simulink model "controller_dev_sg_HIL_noTP"  (R2018b)
settings: configuration reference "Physics" (kept outside this file)
model workspace (MAT data in the model file):
  m = 1000
values from neighbouring files (symbols this model uses):
  bool_activate_Vehicles : value not decoded    [controller_dev_sg.sldd]
  ModObj_ObjList_SendPort = 11004.0    [UDPPortConfig.sldd]
  ModSens_GpsSenDat_SendPort = 3002.0    [UDPPortConfig.sldd]
  sensors_freq_camera = 37.0    [controller_dev_sg.sldd]
  sensors_freq_gps = 20.0    [controller_dev_sg.sldd]
  sensors_freq_imu = 100.0    [controller_dev_sg.sldd]
  sensors_freq_lidar = 12.0    [controller_dev_sg.sldd]
  sensors_freq_radar = 20.0    [controller_dev_sg.sldd]
undefined symbols (not defined in the file or in its folder): activate_VariableFriction, C, tpa_map_Reference, tSPhysics, x0_vehiclepos_start_veh1, x0_vehiclepos_start_veh10, x0_vehiclepos_start_veh2, x0_vehiclepos_start_veh3, x0_vehiclepos_start_veh4, x0_vehiclepos_start_veh5, x0_vehiclepos_start_veh6, x0_vehiclepos_start_veh7, x0_vehiclepos_start_veh8, x0_vehiclepos_start_veh9
libraries: xpcutilitieslib x273, xpcrtudplib x215, aerolibconvert2 x48, simulink x30, etargetslib x26, speedgoatlib_IO612 x7, canmsglib x6, slrtlib x4
(part 5 of 16)

== system controller_dev_sg_HIL_noTP/EnvironmentSim_Communication/prepare data for sending5 ==
  In1 : Inport
  Add : Sum
  Add1 : Sum
  Add2 : Sum
  Bus Selector1 : BusSelector  OutputSignals=x_m,y_m,z_m,phi_rad,theta_rad,psi_rad,nWheelFL_radps,DeltaWheel_rad,nWheelFR_radps,DeltaWheel_rad,nWheelRR_radps,nWheelRL_radps,ax_mps2,ay_mps2,az_mps2,dPhi_radps,dTheta_radps,dPsi_radps,x_m,y_m,psi_rad,vx_mps,vy_mps,nWheelFL_radps,nWheelFR_radps,nWheelRR_radps,nWheelRL_radps
  Clock : Clock
  Constant{,1..5} (6 alike) : Constant  Value=0
  Constant6 : Constant
  Constant7 : Constant  Value=pi
  Constant8 : Constant  Value=pi
  Gain : Gain  Gain=0.5
  Gain1 : Gain  Gain=0.5
  Integrator{,1..3} (4 alike) : Integrator
  Math Function : Math  Operator=square  SaturateOnIntegerOverflow=on
  Math Function1 : Math  Operator=square  SaturateOnIntegerOverflow=on
  Mux : Mux  Inputs=34
  Rate Transition{,1..26} (27 alike) : RateTransition
  Sqrt : Sqrt  SaturateOnIntegerOverflow=on
  normalieAngle1 : MATLAB Function  TreatAsAtomicUnit=on
  normalieAngle2 : MATLAB Function  TreatAsAtomicUnit=on
  Out1 : Outport
  wires:
  In1/1 -> Bus Selector1/1
  Bus Selector1/12 -> Integrator3/1  "<nWheelRL_radps>"
  Gain1/1 -> Add1/1
  Gain/1 -> Add2/2
  Bus Selector1/15 -> Rate Transition14/1  "<az_mps2>"
  Rate Transition22/1 -> Mux/31
  Constant7/1 -> Gain/1
  Bus Selector1/8 -> Rate Transition9/1  "<DeltaWheel_rad>"
  Bus Selector1/22 -> Math Function1/1  "<vx_mps>"
  Rate Transition12/1 -> Mux/20
  Rate Transition13/1 -> Mux/21
  Rate Transition17/1 -> Mux/25
  Sqrt/1 -> Rate Transition21/1
  Constant5/1 -> Mux/8
  Add1/1 -> normalieAngle2/1(u)
  Math Function1/1 -> Add/1
  Constant8/1 -> Gain1/1
  Rate Transition14/1 -> Mux/22
  Math Function/1 -> Add/2
  Bus Selector1/9 -> Integrator1/1  "<nWheelFR_radps>"
  Clock/1 -> Rate Transition26/1
  normalieAngle1/1(y) -> Rate Transition20/1
  Constant4/1 -> Mux/11
  Add2/1 -> normalieAngle1/1(u)
  Constant2/1 -> Mux/16
  Bus Selector1/6 -> Add1/2  "<psi_rad>"
  Constant6/1 -> Mux/29
  Rate Transition20/1 -> Mux/28
  Bus Selector1/24 -> Rate Transition22/1  "<nWheelFL_radps>"
  Integrator2/1 -> Rate Transition10/1
  Add/1 -> Sqrt/1
  Rate Transition23/1 -> Mux/32
  Rate Transition18/1 -> Mux/26
  Rate Transition26/1 -> Mux/1
  Rate Transition25/1 -> Mux/34
  Rate Transition8/1 -> Mux/13
  Bus Selector1/23 -> Math Function/1  "<vy_mps>"
  Bus Selector1/25 -> Rate Transition23/1  "<nWheelFR_radps>"
  Rate Transition10/1 -> Mux/15
  Constant/1 -> Mux/19
  Bus Selector1/20 -> Rate Transition19/1  "<y_m>"
  Rate Transition19/1 -> Mux/27
  Constant3/1 -> Mux/14
  Bus Selector1/21 -> Add2/1  "<psi_rad>"
  Integrator1/1 -> Rate Transition7/1
  Bus Selector1/26 -> Rate Transition24/1  "<nWheelRR_radps>"
  Rate Transition9/1 -> Mux/10
  Bus Selector1/18 -> Rate Transition17/1  "<dPsi_radps>"
  Bus Selector1/19 -> Rate Transition18/1  "<x_m>"
  Bus Selector1/13 -> Rate Transition12/1  "<ax_mps2>"
  Bus Selector1/17 -> Rate Transition16/1  "<dTheta_radps>"
  Integrator3/1 -> Rate Transition11/1
  Rate Transition15/1 -> Mux/23
  Rate Transition2/1 -> Mux/7
  Rate Transition16/1 -> Mux/24
  Bus Selector1/16 -> Rate Transition15/1  "<dPhi_radps>"
  Rate Transition6/1 -> Mux/9
  Rate Transition7/1 -> Mux/12
  Bus Selector1/11 -> Integrator2/1  "<nWheelRR_radps>"
  normalieAngle2/1(y) -> Rate Transition2/1
  Bus Selector1/27 -> Rate Transition25/1  "<nWheelRL_radps>"
  Rate Transition11/1 -> Mux/18
  Bus Selector1/14 -> Rate Transition13/1  "<ay_mps2>"
  Constant1/1 -> Mux/17
  Rate Transition5/1 -> Mux/4
  Rate Transition1/1 -> Mux/3
  Bus Selector1/3 -> Rate Transition5/1  "<z_m>"
  Bus Selector1/5 -> Rate Transition3/1  "<theta_rad>"
  Bus Selector1/2 -> Rate Transition1/1  "<y_m>"
  Bus Selector1/10 -> Rate Transition8/1  "<DeltaWheel_rad>"
  Bus Selector1/7 -> Integrator/1  "<nWheelFL_radps>"
  Bus Selector1/1 -> Rate Transition/1  "<x_m>"
  Integrator/1 -> Rate Transition6/1
  Rate Transition3/1 -> Mux/6
  Bus Selector1/4 -> Rate Transition4/1  "<phi_rad>"
  Rate Transition4/1 -> Mux/5
  Rate Transition21/1 -> Mux/30
  Rate Transition24/1 -> Mux/33
  Rate Transition/1 -> Mux/2
  Mux/1 -> Out1/1

== system controller_dev_sg_HIL_noTP/EnvironmentSim_Communication/prepare data for sending6 ==
  In1 : Inport
  Add : Sum
  Add1 : Sum
  Add2 : Sum
  Bus Selector1 : BusSelector  OutputSignals=x_m,y_m,z_m,phi_rad,theta_rad,psi_rad,nWheelFL_radps,DeltaWheel_rad,nWheelFR_radps,DeltaWheel_rad,nWheelRR_radps,nWheelRL_radps,ax_mps2,ay_mps2,az_mps2,dPhi_radps,dTheta_radps,dPsi_radps,x_m,y_m,psi_rad,vx_mps,vy_mps,nWheelFL_radps,nWheelFR_radps,nWheelRR_radps,nWheelRL_radps
  Clock : Clock
  Constant{,1..5} (6 alike) : Constant  Value=0
  Constant6 : Constant
  Constant7 : Constant  Value=pi
  Constant8 : Constant  Value=pi
  Gain : Gain  Gain=0.5
  Gain1 : Gain  Gain=0.5
  Integrator{,1..3} (4 alike) : Integrator
  Math Function : Math  Operator=square  SaturateOnIntegerOverflow=on
  Math Function1 : Math  Operator=square  SaturateOnIntegerOverflow=on
  Mux : Mux  Inputs=34
  Rate Transition{,1..26} (27 alike) : RateTransition
  Sqrt : Sqrt  SaturateOnIntegerOverflow=on
  normalieAngle1 : MATLAB Function  TreatAsAtomicUnit=on
  normalieAngle2 : MATLAB Function  TreatAsAtomicUnit=on
  Out1 : Outport
  wires:
  In1/1 -> Bus Selector1/1
  Bus Selector1/12 -> Integrator3/1  "<nWheelRL_radps>"
  Gain1/1 -> Add1/1
  Gain/1 -> Add2/2
  Bus Selector1/15 -> Rate Transition14/1  "<az_mps2>"
  Rate Transition22/1 -> Mux/31
  Constant7/1 -> Gain/1
  Bus Selector1/8 -> Rate Transition9/1  "<DeltaWheel_rad>"
  Bus Selector1/22 -> Math Function1/1  "<vx_mps>"
  Rate Transition12/1 -> Mux/20
  Rate Transition13/1 -> Mux/21
  Rate Transition17/1 -> Mux/25
  Sqrt/1 -> Rate Transition21/1
  Constant5/1 -> Mux/8
  Add1/1 -> normalieAngle2/1(u)
  Math Function1/1 -> Add/1
  Constant8/1 -> Gain1/1
  Rate Transition14/1 -> Mux/22
  Math Function/1 -> Add/2
  Bus Selector1/9 -> Integrator1/1  "<nWheelFR_radps>"
  Clock/1 -> Rate Transition26/1
  normalieAngle1/1(y) -> Rate Transition20/1
  Constant4/1 -> Mux/11
  Add2/1 -> normalieAngle1/1(u)
  Constant2/1 -> Mux/16
  Bus Selector1/6 -> Add1/2  "<psi_rad>"
  Constant6/1 -> Mux/29
  Rate Transition20/1 -> Mux/28
  Bus Selector1/24 -> Rate Transition22/1  "<nWheelFL_radps>"
  Integrator2/1 -> Rate Transition10/1
  Add/1 -> Sqrt/1
  Rate Transition23/1 -> Mux/32
  Rate Transition18/1 -> Mux/26
  Rate Transition26/1 -> Mux/1
  Rate Transition25/1 -> Mux/34
  Rate Transition8/1 -> Mux/13
  Bus Selector1/23 -> Math Function/1  "<vy_mps>"
  Bus Selector1/25 -> Rate Transition23/1  "<nWheelFR_radps>"
  Rate Transition10/1 -> Mux/15
  Constant/1 -> Mux/19
  Bus Selector1/20 -> Rate Transition19/1  "<y_m>"
  Rate Transition19/1 -> Mux/27
  Constant3/1 -> Mux/14
  Bus Selector1/21 -> Add2/1  "<psi_rad>"
  Integrator1/1 -> Rate Transition7/1
  Bus Selector1/26 -> Rate Transition24/1  "<nWheelRR_radps>"
  Rate Transition9/1 -> Mux/10
  Bus Selector1/18 -> Rate Transition17/1  "<dPsi_radps>"
  Bus Selector1/19 -> Rate Transition18/1  "<x_m>"
  Bus Selector1/13 -> Rate Transition12/1  "<ax_mps2>"
  Bus Selector1/17 -> Rate Transition16/1  "<dTheta_radps>"
  Integrator3/1 -> Rate Transition11/1
  Rate Transition15/1 -> Mux/23
  Rate Transition2/1 -> Mux/7
  Rate Transition16/1 -> Mux/24
  Bus Selector1/16 -> Rate Transition15/1  "<dPhi_radps>"
  Rate Transition6/1 -> Mux/9
  Rate Transition7/1 -> Mux/12
  Bus Selector1/11 -> Integrator2/1  "<nWheelRR_radps>"
  normalieAngle2/1(y) -> Rate Transition2/1
  Bus Selector1/27 -> Rate Transition25/1  "<nWheelRL_radps>"
  Rate Transition11/1 -> Mux/18
  Bus Selector1/14 -> Rate Transition13/1  "<ay_mps2>"
  Constant1/1 -> Mux/17
  Rate Transition5/1 -> Mux/4
  Rate Transition1/1 -> Mux/3
  Bus Selector1/3 -> Rate Transition5/1  "<z_m>"
  Bus Selector1/5 -> Rate Transition3/1  "<theta_rad>"
  Bus Selector1/2 -> Rate Transition1/1  "<y_m>"
  Bus Selector1/10 -> Rate Transition8/1  "<DeltaWheel_rad>"
  Bus Selector1/7 -> Integrator/1  "<nWheelFL_radps>"
  Bus Selector1/1 -> Rate Transition/1  "<x_m>"
  Integrator/1 -> Rate Transition6/1
  Rate Transition3/1 -> Mux/6
  Bus Selector1/4 -> Rate Transition4/1  "<phi_rad>"
  Rate Transition4/1 -> Mux/5
  Rate Transition21/1 -> Mux/30
  Rate Transition24/1 -> Mux/33
  Rate Transition/1 -> Mux/2
  Mux/1 -> Out1/1

== system controller_dev_sg_HIL_noTP/EnvironmentSim_Communication/prepare data for sending7 ==
  In1 : Inport
  Add : Sum
  Add1 : Sum
  Add2 : Sum
  Bus Selector1 : BusSelector  OutputSignals=x_m,y_m,z_m,phi_rad,theta_rad,psi_rad,nWheelFL_radps,DeltaWheel_rad,nWheelFR_radps,DeltaWheel_rad,nWheelRR_radps,nWheelRL_radps,ax_mps2,ay_mps2,az_mps2,dPhi_radps,dTheta_radps,dPsi_radps,x_m,y_m,psi_rad,vx_mps,vy_mps,nWheelFL_radps,nWheelFR_radps,nWheelRR_radps,nWheelRL_radps
  Clock : Clock
  Constant{,1..5} (6 alike) : Constant  Value=0
  Constant6 : Constant
  Constant7 : Constant  Value=pi
  Constant8 : Constant  Value=pi
  Gain : Gain  Gain=0.5
  Gain1 : Gain  Gain=0.5
  Integrator{,1..3} (4 alike) : Integrator
  Math Function : Math  Operator=square  SaturateOnIntegerOverflow=on
  Math Function1 : Math  Operator=square  SaturateOnIntegerOverflow=on
  Mux : Mux  Inputs=34
  Rate Transition{,1..26} (27 alike) : RateTransition
  Sqrt : Sqrt  SaturateOnIntegerOverflow=on
  normalieAngle1 : MATLAB Function  TreatAsAtomicUnit=on
  normalieAngle2 : MATLAB Function  TreatAsAtomicUnit=on
  Out1 : Outport
  wires:
  In1/1 -> Bus Selector1/1
  Bus Selector1/12 -> Integrator3/1  "<nWheelRL_radps>"
  Gain1/1 -> Add1/1
  Gain/1 -> Add2/2
  Bus Selector1/15 -> Rate Transition14/1  "<az_mps2>"
  Rate Transition22/1 -> Mux/31
  Constant7/1 -> Gain/1
  Bus Selector1/8 -> Rate Transition9/1  "<DeltaWheel_rad>"
  Bus Selector1/22 -> Math Function1/1  "<vx_mps>"
  Rate Transition12/1 -> Mux/20
  Rate Transition13/1 -> Mux/21
  Rate Transition17/1 -> Mux/25
  Sqrt/1 -> Rate Transition21/1
  Constant5/1 -> Mux/8
  Add1/1 -> normalieAngle2/1(u)
  Math Function1/1 -> Add/1
  Constant8/1 -> Gain1/1
  Rate Transition14/1 -> Mux/22
  Math Function/1 -> Add/2
  Bus Selector1/9 -> Integrator1/1  "<nWheelFR_radps>"
  Clock/1 -> Rate Transition26/1
  normalieAngle1/1(y) -> Rate Transition20/1
  Constant4/1 -> Mux/11
  Add2/1 -> normalieAngle1/1(u)
  Constant2/1 -> Mux/16
  Bus Selector1/6 -> Add1/2  "<psi_rad>"
  Constant6/1 -> Mux/29
  Rate Transition20/1 -> Mux/28
  Bus Selector1/24 -> Rate Transition22/1  "<nWheelFL_radps>"
  Integrator2/1 -> Rate Transition10/1
  Add/1 -> Sqrt/1
  Rate Transition23/1 -> Mux/32
  Rate Transition18/1 -> Mux/26
  Rate Transition26/1 -> Mux/1
  Rate Transition25/1 -> Mux/34
  Rate Transition8/1 -> Mux/13
  Bus Selector1/23 -> Math Function/1  "<vy_mps>"
  Bus Selector1/25 -> Rate Transition23/1  "<nWheelFR_radps>"
  Rate Transition10/1 -> Mux/15
  Constant/1 -> Mux/19
  Bus Selector1/20 -> Rate Transition19/1  "<y_m>"
  Rate Transition19/1 -> Mux/27
  Constant3/1 -> Mux/14
  Bus Selector1/21 -> Add2/1  "<psi_rad>"
  Integrator1/1 -> Rate Transition7/1
  Bus Selector1/26 -> Rate Transition24/1  "<nWheelRR_radps>"
  Rate Transition9/1 -> Mux/10
  Bus Selector1/18 -> Rate Transition17/1  "<dPsi_radps>"
  Bus Selector1/19 -> Rate Transition18/1  "<x_m>"
  Bus Selector1/13 -> Rate Transition12/1  "<ax_mps2>"
  Bus Selector1/17 -> Rate Transition16/1  "<dTheta_radps>"
  Integrator3/1 -> Rate Transition11/1
  Rate Transition15/1 -> Mux/23
  Rate Transition2/1 -> Mux/7
  Rate Transition16/1 -> Mux/24
  Bus Selector1/16 -> Rate Transition15/1  "<dPhi_radps>"
  Rate Transition6/1 -> Mux/9
  Rate Transition7/1 -> Mux/12
  Bus Selector1/11 -> Integrator2/1  "<nWheelRR_radps>"
  normalieAngle2/1(y) -> Rate Transition2/1
  Bus Selector1/27 -> Rate Transition25/1  "<nWheelRL_radps>"
  Rate Transition11/1 -> Mux/18
  Bus Selector1/14 -> Rate Transition13/1  "<ay_mps2>"
  Constant1/1 -> Mux/17
  Rate Transition5/1 -> Mux/4
  Rate Transition1/1 -> Mux/3
  Bus Selector1/3 -> Rate Transition5/1  "<z_m>"
  Bus Selector1/5 -> Rate Transition3/1  "<theta_rad>"
  Bus Selector1/2 -> Rate Transition1/1  "<y_m>"
  Bus Selector1/10 -> Rate Transition8/1  "<DeltaWheel_rad>"
  Bus Selector1/7 -> Integrator/1  "<nWheelFL_radps>"
  Bus Selector1/1 -> Rate Transition/1  "<x_m>"
  Integrator/1 -> Rate Transition6/1
  Rate Transition3/1 -> Mux/6
  Bus Selector1/4 -> Rate Transition4/1  "<phi_rad>"
  Rate Transition4/1 -> Mux/5
  Rate Transition21/1 -> Mux/30
  Rate Transition24/1 -> Mux/33
  Rate Transition/1 -> Mux/2
  Mux/1 -> Out1/1

== system controller_dev_sg_HIL_noTP/EnvironmentSim_Communication/prepare data for sending8 ==
  In1 : Inport
  Add : Sum
  Add1 : Sum
  Add2 : Sum
  Bus Selector1 : BusSelector  OutputSignals=x_m,y_m,z_m,phi_rad,theta_rad,psi_rad,nWheelFL_radps,DeltaWheel_rad,nWheelFR_radps,DeltaWheel_rad,nWheelRR_radps,nWheelRL_radps,ax_mps2,ay_mps2,az_mps2,dPhi_radps,dTheta_radps,dPsi_radps,x_m,y_m,psi_rad,vx_mps,vy_mps,nWheelFL_radps,nWheelFR_radps,nWheelRR_radps,nWheelRL_radps
  Clock : Clock
  Constant{,1..5} (6 alike) : Constant  Value=0
  Constant6 : Constant
  Constant7 : Constant  Value=pi
  Constant8 : Constant  Value=pi
  Gain : Gain  Gain=0.5
  Gain1 : Gain  Gain=0.5
  Integrator{,1..3} (4 alike) : Integrator
  Math Function : Math  Operator=square  SaturateOnIntegerOverflow=on
  Math Function1 : Math  Operator=square  SaturateOnIntegerOverflow=on
  Mux : Mux  Inputs=34
  Rate Transition{,1..26} (27 alike) : RateTransition
  Sqrt : Sqrt  SaturateOnIntegerOverflow=on
  normalieAngle1 : MATLAB Function  TreatAsAtomicUnit=on
  normalieAngle2 : MATLAB Function  TreatAsAtomicUnit=on
  Out1 : Outport
  wires:
  In1/1 -> Bus Selector1/1
  Bus Selector1/12 -> Integrator3/1  "<nWheelRL_radps>"
  Gain1/1 -> Add1/1
  Gain/1 -> Add2/2
  Bus Selector1/15 -> Rate Transition14/1  "<az_mps2>"
  Rate Transition22/1 -> Mux/31
  Constant7/1 -> Gain/1
  Bus Selector1/8 -> Rate Transition9/1  "<DeltaWheel_rad>"
  Bus Selector1/22 -> Math Function1/1  "<vx_mps>"
  Rate Transition12/1 -> Mux/20
  Rate Transition13/1 -> Mux/21
  Rate Transition17/1 -> Mux/25
  Sqrt/1 -> Rate Transition21/1
  Constant5/1 -> Mux/8
  Add1/1 -> normalieAngle2/1(u)
  Math Function1/1 -> Add/1
  Constant8/1 -> Gain1/1
  Rate Transition14/1 -> Mux/22
  Math Function/1 -> Add/2
  Bus Selector1/9 -> Integrator1/1  "<nWheelFR_radps>"
  Clock/1 -> Rate Transition26/1
  normalieAngle1/1(y) -> Rate Transition20/1
  Constant4/1 -> Mux/11
  Add2/1 -> normalieAngle1/1(u)
  Constant2/1 -> Mux/16
  Bus Selector1/6 -> Add1/2  "<psi_rad>"
  Constant6/1 -> Mux/29
  Rate Transition20/1 -> Mux/28
  Bus Selector1/24 -> Rate Transition22/1  "<nWheelFL_radps>"
  Integrator2/1 -> Rate Transition10/1
  Add/1 -> Sqrt/1
  Rate Transition23/1 -> Mux/32
  Rate Transition18/1 -> Mux/26
  Rate Transition26/1 -> Mux/1
  Rate Transition25/1 -> Mux/34
  Rate Transition8/1 -> Mux/13
  Bus Selector1/23 -> Math Function/1  "<vy_mps>"
  Bus Selector1/25 -> Rate Transition23/1  "<nWheelFR_radps>"
  Rate Transition10/1 -> Mux/15
  Constant/1 -> Mux/19
  Bus Selector1/20 -> Rate Transition19/1  "<y_m>"
  Rate Transition19/1 -> Mux/27
  Constant3/1 -> Mux/14
  Bus Selector1/21 -> Add2/1  "<psi_rad>"
  Integrator1/1 -> Rate Transition7/1
  Bus Selector1/26 -> Rate Transition24/1  "<nWheelRR_radps>"
  Rate Transition9/1 -> Mux/10
  Bus Selector1/18 -> Rate Transition17/1  "<dPsi_radps>"
  Bus Selector1/19 -> Rate Transition18/1  "<x_m>"
  Bus Selector1/13 -> Rate Transition12/1  "<ax_mps2>"
  Bus Selector1/17 -> Rate Transition16/1  "<dTheta_radps>"
  Integrator3/1 -> Rate Transition11/1
  Rate Transition15/1 -> Mux/23
  Rate Transition2/1 -> Mux/7
  Rate Transition16/1 -> Mux/24
  Bus Selector1/16 -> Rate Transition15/1  "<dPhi_radps>"
  Rate Transition6/1 -> Mux/9
  Rate Transition7/1 -> Mux/12
  Bus Selector1/11 -> Integrator2/1  "<nWheelRR_radps>"
  normalieAngle2/1(y) -> Rate Transition2/1
  Bus Selector1/27 -> Rate Transition25/1  "<nWheelRL_radps>"
  Rate Transition11/1 -> Mux/18
  Bus Selector1/14 -> Rate Transition13/1  "<ay_mps2>"
  Constant1/1 -> Mux/17
  Rate Transition5/1 -> Mux/4
  Rate Transition1/1 -> Mux/3
  Bus Selector1/3 -> Rate Transition5/1  "<z_m>"
  Bus Selector1/5 -> Rate Transition3/1  "<theta_rad>"
  Bus Selector1/2 -> Rate Transition1/1  "<y_m>"
  Bus Selector1/10 -> Rate Transition8/1  "<DeltaWheel_rad>"
  Bus Selector1/7 -> Integrator/1  "<nWheelFL_radps>"
  Bus Selector1/1 -> Rate Transition/1  "<x_m>"
  Integrator/1 -> Rate Transition6/1
  Rate Transition3/1 -> Mux/6
  Bus Selector1/4 -> Rate Transition4/1  "<phi_rad>"
  Rate Transition4/1 -> Mux/5
  Rate Transition21/1 -> Mux/30
  Rate Transition24/1 -> Mux/33
  Rate Transition/1 -> Mux/2
  Mux/1 -> Out1/1

== system controller_dev_sg_HIL_noTP/EnvironmentSim_Communication/prepare data for sending9 ==
  In1 : Inport
  Add : Sum
  Add1 : Sum
  Add2 : Sum
  Bus Selector1 : BusSelector  OutputSignals=x_m,y_m,z_m,phi_rad,theta_rad,psi_rad,nWheelFL_radps,DeltaWheel_rad,nWheelFR_radps,DeltaWheel_rad,nWheelRR_radps,nWheelRL_radps,ax_mps2,ay_mps2,az_mps2,dPhi_radps,dTheta_radps,dPsi_radps,x_m,y_m,psi_rad,vx_mps,vy_mps,nWheelFL_radps,nWheelFR_radps,nWheelRR_radps,nWheelRL_radps
  Clock : Clock
  Constant{,1..5} (6 alike) : Constant  Value=0
  Constant6 : Constant
  Constant7 : Constant  Value=pi
  Constant8 : Constant  Value=pi
  Gain : Gain  Gain=0.5
  Gain1 : Gain  Gain=0.5
  Integrator{,1..3} (4 alike) : Integrator
  Math Function : Math  Operator=square  SaturateOnIntegerOverflow=on
  Math Function1 : Math  Operator=square  SaturateOnIntegerOverflow=on
  Mux : Mux  Inputs=34
  Rate Transition{,1..26} (27 alike) : RateTransition
  Sqrt : Sqrt  SaturateOnIntegerOverflow=on
  normalieAngle1 : MATLAB Function  TreatAsAtomicUnit=on
  normalieAngle2 : MATLAB Function  TreatAsAtomicUnit=on
  Out1 : Outport
  wires:
  In1/1 -> Bus Selector1/1
  Bus Selector1/12 -> Integrator3/1  "<nWheelRL_radps>"
  Gain1/1 -> Add1/1
  Gain/1 -> Add2/2
  Bus Selector1/15 -> Rate Transition14/1  "<az_mps2>"
  Rate Transition22/1 -> Mux/31
  Constant7/1 -> Gain/1
  Bus Selector1/8 -> Rate Transition9/1  "<DeltaWheel_rad>"
  Bus Selector1/22 -> Math Function1/1  "<vx_mps>"
  Rate Transition12/1 -> Mux/20
  Rate Transition13/1 -> Mux/21
  Rate Transition17/1 -> Mux/25
  Sqrt/1 -> Rate Transition21/1
  Constant5/1 -> Mux/8
  Add1/1 -> normalieAngle2/1(u)
  Math Function1/1 -> Add/1
  Constant8/1 -> Gain1/1
  Rate Transition14/1 -> Mux/22
  Math Function/1 -> Add/2
  Bus Selector1/9 -> Integrator1/1  "<nWheelFR_radps>"
  Clock/1 -> Rate Transition26/1
  normalieAngle1/1(y) -> Rate Transition20/1
  Constant4/1 -> Mux/11
  Add2/1 -> normalieAngle1/1(u)
  Constant2/1 -> Mux/16
  Bus Selector1/6 -> Add1/2  "<psi_rad>"
  Constant6/1 -> Mux/29
  Rate Transition20/1 -> Mux/28
  Bus Selector1/24 -> Rate Transition22/1  "<nWheelFL_radps>"
  Integrator2/1 -> Rate Transition10/1
  Add/1 -> Sqrt/1
  Rate Transition23/1 -> Mux/32
  Rate Transition18/1 -> Mux/26
  Rate Transition26/1 -> Mux/1
  Rate Transition25/1 -> Mux/34
  Rate Transition8/1 -> Mux/13
  Bus Selector1/23 -> Math Function/1  "<vy_mps>"
  Bus Selector1/25 -> Rate Transition23/1  "<nWheelFR_radps>"
  Rate Transition10/1 -> Mux/15
  Constant/1 -> Mux/19
  Bus Selector1/20 -> Rate Transition19/1  "<y_m>"
  Rate Transition19/1 -> Mux/27
  Constant3/1 -> Mux/14
  Bus Selector1/21 -> Add2/1  "<psi_rad>"
  Integrator1/1 -> Rate Transition7/1
  Bus Selector1/26 -> Rate Transition24/1  "<nWheelRR_radps>"
  Rate Transition9/1 -> Mux/10
  Bus Selector1/18 -> Rate Transition17/1  "<dPsi_radps>"
  Bus Selector1/19 -> Rate Transition18/1  "<x_m>"
  Bus Selector1/13 -> Rate Transition12/1  "<ax_mps2>"
  Bus Selector1/17 -> Rate Transition16/1  "<dTheta_radps>"
  Integrator3/1 -> Rate Transition11/1
  Rate Transition15/1 -> Mux/23
  Rate Transition2/1 -> Mux/7
  Rate Transition16/1 -> Mux/24
  Bus Selector1/16 -> Rate Transition15/1  "<dPhi_radps>"
  Rate Transition6/1 -> Mux/9
  Rate Transition7/1 -> Mux/12
  Bus Selector1/11 -> Integrator2/1  "<nWheelRR_radps>"
  normalieAngle2/1(y) -> Rate Transition2/1
  Bus Selector1/27 -> Rate Transition25/1  "<nWheelRL_radps>"
  Rate Transition11/1 -> Mux/18
  Bus Selector1/14 -> Rate Transition13/1  "<ay_mps2>"
  Constant1/1 -> Mux/17
  Rate Transition5/1 -> Mux/4
  Rate Transition1/1 -> Mux/3
  Bus Selector1/3 -> Rate Transition5/1  "<z_m>"
  Bus Selector1/5 -> Rate Transition3/1  "<theta_rad>"
  Bus Selector1/2 -> Rate Transition1/1  "<y_m>"
  Bus Selector1/10 -> Rate Transition8/1  "<DeltaWheel_rad>"
  Bus Selector1/7 -> Integrator/1  "<nWheelFL_radps>"
  Bus Selector1/1 -> Rate Transition/1  "<x_m>"
  Integrator/1 -> Rate Transition6/1
  Rate Transition3/1 -> Mux/6
  Bus Selector1/4 -> Rate Transition4/1  "<phi_rad>"
  Rate Transition4/1 -> Mux/5
  Rate Transition21/1 -> Mux/30
  Rate Transition24/1 -> Mux/33
  Rate Transition/1 -> Mux/2
  Mux/1 -> Out1/1

== system controller_dev_sg_HIL_noTP/Subsystem4/ReadSteeringWheelInput ==
  Compare To Constant : simulink/Logic and Bit Operations/Compare To Constant  Priority=1  relop===  const=24  OutDataTypeStr=boolean
  Min. do-while count : Constant  OutDataTypeStr=int8  SampleTime=-1
  Subtrat : Sum  Inputs=+-
  UDP Receive : xpcrtudplib/UDP Receive  ipAddressVal=192.168.0.2  localPort=50004  rcvWidth=24  rcvFmAny=on  fmAddress=10.0.2.0  rcvMulticast=off  multicastAddress={}  maxUDPQueue=8  sampleTime=-1
      settings: SourceProductName=Simulink Real-Time
  While Iterator : WhileIterator  WhileBlockType=do-while  ShowIterationPort=on  OutputDataType=int16
  NumMsg : Outport
  Data : Outport  Port=2
  wires:
  Subtrat/1 -> NumMsg/1  "num msgs this timestep"
  UDP Receive/1 -> Data/1
  Min. do-while count/1 -> Subtrat/2
  While Iterator/1 -> Subtrat/1
  UDP Receive/2 -> Compare To Constant/1
  Compare To Constant/1 -> While Iterator/1

== system controller_dev_sg_HIL_noTP/Subsystem4/ReadSteeringWheelInputPackage ==
  Raw Data : Inport
  Enable : EnablePort
  Byte Unpack : etargetslib/Byte Unpack  dimensions={[1], [1], [1]}  datatypes={'double', 'double', 'double'}  byteAlign=1
  Terminator : Terminator
  Acceleration : Outport
  SteeringWheelAngle_rad : Outport  Port=2
  wires:
  Byte Unpack/1 -> Acceleration/1
  Byte Unpack/2 -> SteeringWheelAngle_rad/1
  Byte Unpack/3 -> Terminator/1
  Raw Data/1 -> Byte Unpack/1

== system controller_dev_sg_HIL_noTP/UDP from Control (Request for Steering Angle, Long. Force)/ReadControlCommands ==
  Compare To Constant : simulink/Logic and Bit Operations/Compare To Constant  relop===  const=40  OutDataTypeStr=boolean
  Min. do-while count : Constant  OutDataTypeStr=int8  SampleTime=-1
  Subtrat : Sum  Inputs=+-
  UDP Receive : xpcrtudplib/UDP Receive  ipAddressVal=10.0.0.20  localPort=ModCtrl_CtrlCommandVeh1_RcvPort  rcvWidth=40  rcvFmAny=on  fmAddress=10.0.0.1  rcvMulticast=off  multicastAddress={}  maxUDPQueue=8  sampleTime=-1
      settings: SourceProductName=Simulink Real-Time
  While Iterator : WhileIterator  WhileBlockType=do-while  ShowIterationPort=on  OutputDataType=int16
  Data : Outport
  NumMsg : Outport  Port=2
  wires:
  Compare To Constant/1 -> While Iterator/1
  UDP Receive/2 -> Compare To Constant/1
  While Iterator/1 -> Subtrat/1
  Min. do-while count/1 -> Subtrat/2
  Subtrat/1 -> NumMsg/1  "num msgs this timestep"
  UDP Receive/1 -> Data/1

== system controller_dev_sg_HIL_noTP/UDP from Control (Request for Steering Angle, Long. Force)/ReadControlCommandsPackage ==
  Raw Data : Inport
  Enable : EnablePort
  Byte Unpack : etargetslib/Byte Unpack  dimensions={[1], [1], [1], [1], [1]}  datatypes={'double', 'double', 'double', 'double', 'double'}  byteAlign=1
  Data Type Conversion{,1..4} (5 alike) : DataTypeConversion  OutDataTypeStr=double
  SteeringAngleRequest_rad : Outport
  LongForceRequest_N : Outport  Port=2
  ThrottleRequest_perc : Outport  Port=3
  GearRequest : Outport  Port=4
  BrakeRequest_bar : Outport  Port=5
  wires:
  Byte Unpack/1 -> Data Type Conversion/1
  Raw Data/1 -> Byte Unpack/1
  Byte Unpack/2 -> Data Type Conversion1/1
  Data Type Conversion/1 -> SteeringAngleRequest_rad/1
  Data Type Conversion1/1 -> LongForceRequest_N/1
  Byte Unpack/3 -> Data Type Conversion2/1
  Byte Unpack/4 -> Data Type Conversion3/1
  Byte Unpack/5 -> Data Type Conversion4/1
  Data Type Conversion2/1 -> ThrottleRequest_perc/1
  Data Type Conversion3/1 -> GearRequest/1
  Data Type Conversion4/1 -> BrakeRequest_bar/1

== system controller_dev_sg_HIL_noTP/UDP from Control (Request for Steering Angle, Long. Force)1/ReadControlCommands ==
  Compare To Constant : simulink/Logic and Bit Operations/Compare To Constant  relop===  const=40  OutDataTypeStr=boolean
  Min. do-while count : Constant  OutDataTypeStr=int8  SampleTime=-1
  Subtrat : Sum  Inputs=+-
  UDP Receive : xpcrtudplib/UDP Receive  ipAddressVal=10.0.0.20  localPort=ModCtrl_CtrlCommandVeh2_RcvPort  rcvWidth=40  rcvFmAny=on  fmAddress=10.0.0.1  rcvMulticast=off  multicastAddress={}  maxUDPQueue=8  sampleTime=-1
      settings: SourceProductName=Simulink Real-Time
  While Iterator : WhileIterator  WhileBlockType=do-while  ShowIterationPort=on  OutputDataType=int16
  Data : Outport
  NumMsg : Outport  Port=2
  wires:
  Compare To Constant/1 -> While Iterator/1
  UDP Receive/2 -> Compare To Constant/1
  While Iterator/1 -> Subtrat/1
  Min. do-while count/1 -> Subtrat/2
  Subtrat/1 -> NumMsg/1  "num msgs this timestep"
  UDP Receive/1 -> Data/1

== system controller_dev_sg_HIL_noTP/UDP from Control (Request for Steering Angle, Long. Force)1/ReadControlCommandsPackage ==
  Raw Data : Inport
  Enable : EnablePort
  Byte Unpack : etargetslib/Byte Unpack  dimensions={[1], [1], [1], [1], [1]}  datatypes={'double', 'double', 'double', 'double', 'double'}  byteAlign=1
  Data Type Conversion{,1..4} (5 alike) : DataTypeConversion  OutDataTypeStr=double
  SteeringAngleAtWheel_rad : Outport
  TractionForceSummedAtWheels_N : Outport  Port=2
  ThrottleRequest_perc : Outport  Port=3
  GearRequest : Outport  Port=4
  BrakeRequest_bar : Outport  Port=5
  wires:
  Byte Unpack/1 -> Data Type Conversion/1
  Raw Data/1 -> Byte Unpack/1
  Byte Unpack/2 -> Data Type Conversion1/1
  Data Type Conversion2/1 -> ThrottleRequest_perc/1
  Data Type Conversion4/1 -> BrakeRequest_bar/1
  Data Type Conversion/1 -> SteeringAngleAtWheel_rad/1
  Data Type Conversion1/1 -> TractionForceSummedAtWheels_N/1
  Data Type Conversion3/1 -> GearRequest/1
  Byte Unpack/3 -> Data Type Conversion2/1
  Byte Unpack/4 -> Data Type Conversion3/1
  Byte Unpack/5 -> Data Type Conversion4/1

== system controller_dev_sg_HIL_noTP/UDP from Control (Request for Steering Angle, Long. Force)2/ReadControlCommands ==
  Compare To Constant : simulink/Logic and Bit Operations/Compare To Constant  relop===  const=40  OutDataTypeStr=boolean
  Min. do-while count : Constant  OutDataTypeStr=int8  SampleTime=-1
  Subtrat : Sum  Inputs=+-
  UDP Receive : xpcrtudplib/UDP Receive  ipAddressVal=10.0.0.20  localPort=ModCtrl_CtrlCommandVeh3_RcvPort  rcvWidth=40  rcvFmAny=on  fmAddress=10.0.0.1  rcvMulticast=off  multicastAddress={}  maxUDPQueue=8  sampleTime=-1
      settings: SourceProductName=Simulink Real-Time
  While Iterator : WhileIterator  WhileBlockType=do-while  ShowIterationPort=on  OutputDataType=int16
  Data : Outport
  NumMsg : Outport  Port=2
  wires:
  Compare To Constant/1 -> While Iterator/1
  UDP Receive/2 -> Compare To Constant/1
  While Iterator/1 -> Subtrat/1
  Min. do-while count/1 -> Subtrat/2
  Subtrat/1 -> NumMsg/1  "num msgs this timestep"
  UDP Receive/1 -> Data/1

== system controller_dev_sg_HIL_noTP/UDP from Control (Request for Steering Angle, Long. Force)2/ReadControlCommandsPackage ==
  Raw Data : Inport
  Enable : EnablePort
  Byte Unpack : etargetslib/Byte Unpack  dimensions={[1], [1], [1], [1], [1]}  datatypes={'double', 'double', 'double', 'double', 'double'}  byteAlign=1
  Data Type Conversion{,1..2,4..5} (5 alike) : DataTypeConversion  OutDataTypeStr=double
  SteeringAngleAtWheel_rad : Outport
  TractionForceSummedAtWheels_N : Outport  Port=2
  ThrottleRequest_perc : Outport  Port=3
  GearRequest : Outport  Port=4
  BrakeRequest_bar : Outport  Port=5
  wires:
  Byte Unpack/1 -> Data Type Conversion/1
  Raw Data/1 -> Byte Unpack/1
  Byte Unpack/2 -> Data Type Conversion1/1
  Data Type Conversion2/1 -> ThrottleRequest_perc/1
  Data Type Conversion5/1 -> BrakeRequest_bar/1
  Data Type Conversion/1 -> SteeringAngleAtWheel_rad/1
  Data Type Conversion1/1 -> TractionForceSummedAtWheels_N/1
  Data Type Conversion4/1 -> GearRequest/1
  Byte Unpack/5 -> Data Type Conversion5/1
  Byte Unpack/4 -> Data Type Conversion4/1
  Byte Unpack/3 -> Data Type Conversion2/1

== system controller_dev_sg_HIL_noTP/UDP from Control (Request for Steering Angle, Long. Force)3/ReadControlCommands ==
  Compare To Constant : simulink/Logic and Bit Operations/Compare To Constant  relop===  const=40  OutDataTypeStr=boolean
  Min. do-while count : Constant  OutDataTypeStr=int8  SampleTime=-1
  Subtrat : Sum  Inputs=+-
  UDP Receive : xpcrtudplib/UDP Receive  ipAddressVal=10.0.0.20  localPort=ModCtrl_CtrlCommandVeh5_RcvPort  rcvWidth=40  rcvFmAny=on  fmAddress=10.0.0.1  rcvMulticast=off  multicastAddress={}  maxUDPQueue=8  sampleTime=-1
      settings: SourceProductName=Simulink Real-Time
  While Iterator : WhileIterator  WhileBlockType=do-while  ShowIterationPort=on  OutputDataType=int16
  Data : Outport
  NumMsg : Outport  Port=2
  wires:
  Compare To Constant/1 -> While Iterator/1
  UDP Receive/2 -> Compare To Constant/1
  While Iterator/1 -> Subtrat/1
  Min. do-while count/1 -> Subtrat/2
  Subtrat/1 -> NumMsg/1  "num msgs this timestep"
  UDP Receive/1 -> Data/1

== system controller_dev_sg_HIL_noTP/UDP from Control (Request for Steering Angle, Long. Force)3/ReadControlCommandsPackage ==
  Raw Data : Inport
  Enable : EnablePort
  Byte Unpack : etargetslib/Byte Unpack  dimensions={[1], [1], [1], [1], [1]}  datatypes={'double', 'double', 'double', 'double', 'double'}  byteAlign=1
  Data Type Conversion{,1..4} (5 alike) : DataTypeConversion  OutDataTypeStr=double
  SteeringAngleAtWheel_rad : Outport
  TractionForceSummedAtWheels_N : Outport  Port=2
  ThrottleRequest_perc : Outport  Port=3
  GearRequest : Outport  Port=4
  BrakeRequest_bar : Outport  Port=5
  wires:
  Byte Unpack/1 -> Data Type Conversion/1
  Raw Data/1 -> Byte Unpack/1
  Byte Unpack/2 -> Data Type Conversion1/1
  Byte Unpack/5 -> Data Type Conversion4/1
  Byte Unpack/4 -> Data Type Conversion3/1
  Byte Unpack/3 -> Data Type Conversion2/1
  Data Type Conversion2/1 -> ThrottleRequest_perc/1
  Data Type Conversion/1 -> SteeringAngleAtWheel_rad/1
  Data Type Conversion4/1 -> BrakeRequest_bar/1
  Data Type Conversion3/1 -> GearRequest/1
  Data Type Conversion1/1 -> TractionForceSummedAtWheels_N/1

== system controller_dev_sg_HIL_noTP/UDP from Control (Request for Steering Angle, Long. Force)4/ReadControlCommands ==
  Compare To Constant : simulink/Logic and Bit Operations/Compare To Constant  relop===  const=40  OutDataTypeStr=boolean
  Min. do-while count : Constant  OutDataTypeStr=int8  SampleTime=-1
  Subtrat : Sum  Inputs=+-
  UDP Receive : xpcrtudplib/UDP Receive  ipAddressVal=10.0.0.20  localPort=ModCtrl_CtrlCommandVeh4_RcvPort  rcvWidth=40  rcvFmAny=on  fmAddress=10.0.0.1  rcvMulticast=off  multicastAddress={}  maxUDPQueue=8  sampleTime=-1
      settings: SourceProductName=Simulink Real-Time
  While Iterator : WhileIterator  WhileBlockType=do-while  ShowIterationPort=on  OutputDataType=int16
  Data : Outport
  NumMsg : Outport  Port=2
  wires:
  Compare To Constant/1 -> While Iterator/1
  UDP Receive/2 -> Compare To Constant/1
  While Iterator/1 -> Subtrat/1
  Min. do-while count/1 -> Subtrat/2
  Subtrat/1 -> NumMsg/1  "num msgs this timestep"
  UDP Receive/1 -> Data/1

== system controller_dev_sg_HIL_noTP/UDP from Control (Request for Steering Angle, Long. Force)4/ReadControlCommandsPackage ==
  Raw Data : Inport
  Enable : EnablePort
  Byte Unpack : etargetslib/Byte Unpack  dimensions={[1], [1], [1], [1], [1]}  datatypes={'double', 'double', 'double', 'double', 'double'}  byteAlign=1
  Data Type Conversion{,1..4} (5 alike) : DataTypeConversion  OutDataTypeStr=double
  SteeringAngleAtWheel_rad : Outport
  TractionForceSummedAtWheels_N : Outport  Port=2
  ThrottleRequest_perc : Outport  Port=3
  GearRequest : Outport  Port=4
  BrakeRequest_bar : Outport  Port=5
  wires:
  Byte Unpack/1 -> Data Type Conversion/1
  Raw Data/1 -> Byte Unpack/1
  Byte Unpack/2 -> Data Type Conversion1/1
  Byte Unpack/5 -> Data Type Conversion4/1
  Byte Unpack/4 -> Data Type Conversion3/1
  Byte Unpack/3 -> Data Type Conversion2/1
  Data Type Conversion2/1 -> ThrottleRequest_perc/1
  Data Type Conversion/1 -> SteeringAngleAtWheel_rad/1
  Data Type Conversion4/1 -> BrakeRequest_bar/1
  Data Type Conversion3/1 -> GearRequest/1
  Data Type Conversion1/1 -> TractionForceSummedAtWheels_N/1

== system controller_dev_sg_HIL_noTP/UDP from Control (Request for Steering Angle, Long. Force)5/ReadControlCommands ==
  Compare To Constant : simulink/Logic and Bit Operations/Compare To Constant  relop===  const=40  OutDataTypeStr=boolean
  Min. do-while count : Constant  OutDataTypeStr=int8  SampleTime=-1
  Subtrat : Sum  Inputs=+-
  UDP Receive : xpcrtudplib/UDP Receive  ipAddressVal=10.0.0.20  localPort=ModCtrl_CtrlCommandVeh6_RcvPort  rcvWidth=40  rcvFmAny=on  fmAddress=10.0.0.1  rcvMulticast=off  multicastAddress={}  maxUDPQueue=8  sampleTime=-1
      settings: SourceProductName=Simulink Real-Time
  While Iterator : WhileIterator  WhileBlockType=do-while  ShowIterationPort=on  OutputDataType=int16
  Data : Outport
  NumMsg : Outport  Port=2
  wires:
  Compare To Constant/1 -> While Iterator/1
  UDP Receive/2 -> Compare To Constant/1
  While Iterator/1 -> Subtrat/1
  Min. do-while count/1 -> Subtrat/2
  Subtrat/1 -> NumMsg/1  "num msgs this timestep"
  UDP Receive/1 -> Data/1

== system controller_dev_sg_HIL_noTP/UDP from Control (Request for Steering Angle, Long. Force)5/ReadControlCommandsPackage ==
  Raw Data : Inport
  Enable : EnablePort
  Byte Unpack : etargetslib/Byte Unpack  dimensions={[1], [1], [1], [1], [1]}  datatypes={'double', 'double', 'double', 'double', 'double'}  byteAlign=1
  Data Type Conversion{,1..4} (5 alike) : DataTypeConversion  OutDataTypeStr=double
  SteeringAngleAtWheel_rad : Outport
  TractionForceSummedAtWheels_N : Outport  Port=2
  ThrottleRequest_perc : Outport  Port=3
  GearRequest : Outport  Port=4
  BrakeRequest_bar : Outport  Port=5
  wires:
  Byte Unpack/1 -> Data Type Conversion/1
  Raw Data/1 -> Byte Unpack/1
  Byte Unpack/2 -> Data Type Conversion1/1
  Byte Unpack/5 -> Data Type Conversion4/1
  Byte Unpack/4 -> Data Type Conversion3/1
  Byte Unpack/3 -> Data Type Conversion2/1
  Data Type Conversion2/1 -> ThrottleRequest_perc/1
  Data Type Conversion/1 -> SteeringAngleAtWheel_rad/1
  Data Type Conversion4/1 -> BrakeRequest_bar/1
  Data Type Conversion3/1 -> GearRequest/1
  Data Type Conversion1/1 -> TractionForceSummedAtWheels_N/1

== system controller_dev_sg_HIL_noTP/UDP from Control (Request for Steering Angle, Long. Force)6/ReadControlCommands ==
  Compare To Constant : simulink/Logic and Bit Operations/Compare To Constant  relop===  const=40  OutDataTypeStr=boolean
  Min. do-while count : Constant  OutDataTypeStr=int8  SampleTime=-1
  Subtrat : Sum  Inputs=+-
  UDP Receive : xpcrtudplib/UDP Receive  ipAddressVal=10.0.0.20  localPort=ModCtrl_CtrlCommandVeh7_RcvPort  rcvWidth=40  rcvFmAny=on  fmAddress=10.0.0.1  rcvMulticast=off  multicastAddress={}  maxUDPQueue=8  sampleTime=-1
      settings: SourceProductName=Simulink Real-Time
  While Iterator : WhileIterator  WhileBlockType=do-while  ShowIterationPort=on  OutputDataType=int16
  Data : Outport
  NumMsg : Outport  Port=2
  wires:
  Compare To Constant/1 -> While Iterator/1
  UDP Receive/2 -> Compare To Constant/1
  While Iterator/1 -> Subtrat/1
  Min. do-while count/1 -> Subtrat/2
  Subtrat/1 -> NumMsg/1  "num msgs this timestep"
  UDP Receive/1 -> Data/1

== system controller_dev_sg_HIL_noTP/UDP from Control (Request for Steering Angle, Long. Force)6/ReadControlCommandsPackage ==
  Raw Data : Inport
  Enable : EnablePort
  Byte Unpack : etargetslib/Byte Unpack  dimensions={[1], [1], [1], [1], [1]}  datatypes={'double', 'double', 'double', 'double', 'double'}  byteAlign=1
  Data Type Conversion{,1..4} (5 alike) : DataTypeConversion  OutDataTypeStr=double
  SteeringAngleAtWheel_rad : Outport
  TractionForceSummedAtWheels_N : Outport  Port=2
  ThrottleRequest_perc : Outport  Port=3
  GearRequest : Outport  Port=4
  BrakeRequest_bar : Outport  Port=5
  wires:
  Byte Unpack/1 -> Data Type Conversion/1
  Raw Data/1 -> Byte Unpack/1
  Byte Unpack/2 -> Data Type Conversion1/1
  Byte Unpack/5 -> Data Type Conversion4/1
  Byte Unpack/4 -> Data Type Conversion3/1
  Byte Unpack/3 -> Data Type Conversion2/1
  Data Type Conversion2/1 -> ThrottleRequest_perc/1
  Data Type Conversion/1 -> SteeringAngleAtWheel_rad/1
  Data Type Conversion4/1 -> BrakeRequest_bar/1
  Data Type Conversion3/1 -> GearRequest/1
  Data Type Conversion1/1 -> TractionForceSummedAtWheels_N/1

== system controller_dev_sg_HIL_noTP/UDP from Control (Request for Steering Angle, Long. Force)7/ReadControlCommands ==
  Compare To Constant : simulink/Logic and Bit Operations/Compare To Constant  relop===  const=40  OutDataTypeStr=boolean
  Min. do-while count : Constant  OutDataTypeStr=int8  SampleTime=-1
  Subtrat : Sum  Inputs=+-
  UDP Receive : xpcrtudplib/UDP Receive  ipAddressVal=10.0.0.20  localPort=ModCtrl_CtrlCommandVeh8_RcvPort  rcvWidth=40  rcvFmAny=on  fmAddress=10.0.0.1  rcvMulticast=off  multicastAddress={}  maxUDPQueue=8  sampleTime=-1
      settings: SourceProductName=Simulink Real-Time
  While Iterator : WhileIterator  WhileBlockType=do-while  ShowIterationPort=on  OutputDataType=int16
  Data : Outport
  NumMsg : Outport  Port=2
  wires:
  Compare To Constant/1 -> While Iterator/1
  UDP Receive/2 -> Compare To Constant/1
  While Iterator/1 -> Subtrat/1
  Min. do-while count/1 -> Subtrat/2
  Subtrat/1 -> NumMsg/1  "num msgs this timestep"
  UDP Receive/1 -> Data/1

== system controller_dev_sg_HIL_noTP/UDP from Control (Request for Steering Angle, Long. Force)7/ReadControlCommandsPackage ==
  Raw Data : Inport
  Enable : EnablePort
  Byte Unpack : etargetslib/Byte Unpack  dimensions={[1], [1], [1], [1], [1]}  datatypes={'double', 'double', 'double', 'double', 'double'}  byteAlign=1
  Data Type Conversion{,1..4} (5 alike) : DataTypeConversion  OutDataTypeStr=double
  SteeringAngleAtWheel_rad : Outport
  TractionForceSummedAtWheels_N : Outport  Port=2
  ThrottleRequest_perc : Outport  Port=3
  GearRequest : Outport  Port=4
  BrakeRequest_bar : Outport  Port=5
  wires:
  Byte Unpack/1 -> Data Type Conversion/1
  Raw Data/1 -> Byte Unpack/1
  Byte Unpack/2 -> Data Type Conversion1/1
  Byte Unpack/5 -> Data Type Conversion4/1
  Byte Unpack/4 -> Data Type Conversion3/1
  Byte Unpack/3 -> Data Type Conversion2/1
  Data Type Conversion2/1 -> ThrottleRequest_perc/1
  Data Type Conversion/1 -> SteeringAngleAtWheel_rad/1
  Data Type Conversion4/1 -> BrakeRequest_bar/1
  Data Type Conversion3/1 -> GearRequest/1
  Data Type Conversion1/1 -> TractionForceSummedAtWheels_N/1

== system controller_dev_sg_HIL_noTP/UDP to Object Detection/Prepare Object List1 ==
  Objects : Inport
  Bus Selector1 : BusSelector  OutputSignals=Object_1,Object_2,Object_3,Object_4,Object_5,Object_6,Object_7,Object_8,Object_9,Object_10
  Byte Pack : etargetslib/Byte Pack  datatypes={['double']}  byteAlign=1
  Data Type Conversion4 : DataTypeConversion
  Matrix Concatenate : Concatenate  NumInputs=10  Mode=Multidimensional array
  ObjList_Package : Outport
  wires:
  Byte Pack/1 -> ObjList_Package/1
  Data Type Conversion4/1 -> Byte Pack/1
  Objects/1 -> Bus Selector1/1
  Matrix Concatenate/1 -> Data Type Conversion4/1
  Bus Selector1/1 -> Matrix Concatenate/1  "<Object_1>"
  Bus Selector1/2 -> Matrix Concatenate/2  "<Object_2>"
  Bus Selector1/3 -> Matrix Concatenate/3  "<Object_3>"
  Bus Selector1/4 -> Matrix Concatenate/4  "<Object_4>"
  Bus Selector1/5 -> Matrix Concatenate/5  "<Object_5>"
  Bus Selector1/6 -> Matrix Concatenate/6  "<Object_6>"
  Bus Selector1/7 -> Matrix Concatenate/7  "<Object_7>"
  Bus Selector1/8 -> Matrix Concatenate/8  "<Object_8>"
  Bus Selector1/9 -> Matrix Concatenate/9  "<Object_9>"
  Bus Selector1/10 -> Matrix Concatenate/10  "<Object_10>"

== system controller_dev_sg_HIL_noTP/UDP to Object Detection/Prepare Object List10 ==
  Objects : Inport
  Bus Selector1 : BusSelector  OutputSignals=Object_1,Object_2,Object_3,Object_4,Object_5,Object_6,Object_7,Object_8,Object_9,Object_10
  Byte Pack : etargetslib/Byte Pack  datatypes={['double']}  byteAlign=1
  Data Type Conversion4 : DataTypeConversion
  Matrix Concatenate : Concatenate  NumInputs=10  Mode=Multidimensional array
  ObjList_Package : Outport
  wires:
  Byte Pack/1 -> ObjList_Package/1
  Data Type Conversion4/1 -> Byte Pack/1
  Objects/1 -> Bus Selector1/1
  Matrix Concatenate/1 -> Data Type Conversion4/1
  Bus Selector1/1 -> Matrix Concatenate/1  "<Object_1>"
  Bus Selector1/2 -> Matrix Concatenate/2  "<Object_2>"
  Bus Selector1/3 -> Matrix Concatenate/3  "<Object_3>"
  Bus Selector1/4 -> Matrix Concatenate/4  "<Object_4>"
  Bus Selector1/5 -> Matrix Concatenate/5  "<Object_5>"
  Bus Selector1/6 -> Matrix Concatenate/6  "<Object_6>"
  Bus Selector1/7 -> Matrix Concatenate/7  "<Object_7>"
  Bus Selector1/8 -> Matrix Concatenate/8  "<Object_8>"
  Bus Selector1/9 -> Matrix Concatenate/9  "<Object_9>"
  Bus Selector1/10 -> Matrix Concatenate/10  "<Object_10>"

== system controller_dev_sg_HIL_noTP/UDP to Object Detection/Prepare Object List2 ==
  Objects : Inport
  Bus Selector1 : BusSelector  OutputSignals=Object_1,Object_2,Object_3,Object_4,Object_5,Object_6,Object_7,Object_8,Object_9,Object_10
  Byte Pack : etargetslib/Byte Pack  datatypes={['double']}  byteAlign=1
  Data Type Conversion4 : DataTypeConversion
  Matrix Concatenate : Concatenate  NumInputs=10  Mode=Multidimensional array
  ObjList_Package : Outport
  wires:
  Byte Pack/1 -> ObjList_Package/1
  Data Type Conversion4/1 -> Byte Pack/1
  Objects/1 -> Bus Selector1/1
  Matrix Concatenate/1 -> Data Type Conversion4/1
  Bus Selector1/1 -> Matrix Concatenate/1  "<Object_1>"
  Bus Selector1/2 -> Matrix Concatenate/2  "<Object_2>"
  Bus Selector1/3 -> Matrix Concatenate/3  "<Object_3>"
  Bus Selector1/4 -> Matrix Concatenate/4  "<Object_4>"
  Bus Selector1/5 -> Matrix Concatenate/5  "<Object_5>"
  Bus Selector1/6 -> Matrix Concatenate/6  "<Object_6>"
  Bus Selector1/7 -> Matrix Concatenate/7  "<Object_7>"
  Bus Selector1/8 -> Matrix Concatenate/8  "<Object_8>"
  Bus Selector1/9 -> Matrix Concatenate/9  "<Object_9>"
  Bus Selector1/10 -> Matrix Concatenate/10  "<Object_10>"

== system controller_dev_sg_HIL_noTP/UDP to Object Detection/Prepare Object List3 ==
  Objects : Inport
  Bus Selector1 : BusSelector  OutputSignals=Object_1,Object_2,Object_3,Object_4,Object_5,Object_6,Object_7,Object_8,Object_9,Object_10
  Byte Pack : etargetslib/Byte Pack  datatypes={['double']}  byteAlign=1
  Data Type Conversion4 : DataTypeConversion
  Matrix Concatenate : Concatenate  NumInputs=10  Mode=Multidimensional array
  ObjList_Package : Outport
  wires:
  Byte Pack/1 -> ObjList_Package/1
  Data Type Conversion4/1 -> Byte Pack/1
  Objects/1 -> Bus Selector1/1
  Matrix Concatenate/1 -> Data Type Conversion4/1
  Bus Selector1/1 -> Matrix Concatenate/1  "<Object_1>"
  Bus Selector1/2 -> Matrix Concatenate/2  "<Object_2>"
  Bus Selector1/3 -> Matrix Concatenate/3  "<Object_3>"
  Bus Selector1/4 -> Matrix Concatenate/4  "<Object_4>"
  Bus Selector1/5 -> Matrix Concatenate/5  "<Object_5>"
  Bus Selector1/6 -> Matrix Concatenate/6  "<Object_6>"
  Bus Selector1/7 -> Matrix Concatenate/7  "<Object_7>"
  Bus Selector1/8 -> Matrix Concatenate/8  "<Object_8>"
  Bus Selector1/9 -> Matrix Concatenate/9  "<Object_9>"
  Bus Selector1/10 -> Matrix Concatenate/10  "<Object_10>"

== system controller_dev_sg_HIL_noTP/UDP to Object Detection/Prepare Object List4 ==
  Objects : Inport
  Bus Selector1 : BusSelector  OutputSignals=Object_1,Object_2,Object_3,Object_4,Object_5,Object_6,Object_7,Object_8,Object_9,Object_10
  Byte Pack : etargetslib/Byte Pack  datatypes={['double']}  byteAlign=1
  Data Type Conversion4 : DataTypeConversion
  Matrix Concatenate : Concatenate  NumInputs=10  Mode=Multidimensional array
  ObjList_Package : Outport
  wires:
  Byte Pack/1 -> ObjList_Package/1
  Data Type Conversion4/1 -> Byte Pack/1
  Objects/1 -> Bus Selector1/1
  Matrix Concatenate/1 -> Data Type Conversion4/1
  Bus Selector1/1 -> Matrix Concatenate/1  "<Object_1>"
  Bus Selector1/2 -> Matrix Concatenate/2  "<Object_2>"
  Bus Selector1/3 -> Matrix Concatenate/3  "<Object_3>"
  Bus Selector1/4 -> Matrix Concatenate/4  "<Object_4>"
  Bus Selector1/5 -> Matrix Concatenate/5  "<Object_5>"
  Bus Selector1/6 -> Matrix Concatenate/6  "<Object_6>"
  Bus Selector1/7 -> Matrix Concatenate/7  "<Object_7>"
  Bus Selector1/8 -> Matrix Concatenate/8  "<Object_8>"
  Bus Selector1/9 -> Matrix Concatenate/9  "<Object_9>"
  Bus Selector1/10 -> Matrix Concatenate/10  "<Object_10>"

== system controller_dev_sg_HIL_noTP/UDP to Object Detection/Prepare Object List5 ==
  Objects : Inport
  Bus Selector1 : BusSelector  OutputSignals=Object_1,Object_2,Object_3,Object_4,Object_5,Object_6,Object_7,Object_8,Object_9,Object_10
  Byte Pack : etargetslib/Byte Pack  datatypes={['double']}  byteAlign=1
  Data Type Conversion4 : DataTypeConversion
  Matrix Concatenate : Concatenate  NumInputs=10  Mode=Multidimensional array
  ObjList_Package : Outport
  wires:
  Byte Pack/1 -> ObjList_Package/1
  Data Type Conversion4/1 -> Byte Pack/1
  Objects/1 -> Bus Selector1/1
  Matrix Concatenate/1 -> Data Type Conversion4/1
  Bus Selector1/1 -> Matrix Concatenate/1  "<Object_1>"
  Bus Selector1/2 -> Matrix Concatenate/2  "<Object_2>"
  Bus Selector1/3 -> Matrix Concatenate/3  "<Object_3>"
  Bus Selector1/4 -> Matrix Concatenate/4  "<Object_4>"
  Bus Selector1/5 -> Matrix Concatenate/5  "<Object_5>"
  Bus Selector1/6 -> Matrix Concatenate/6  "<Object_6>"
  Bus Selector1/7 -> Matrix Concatenate/7  "<Object_7>"
  Bus Selector1/8 -> Matrix Concatenate/8  "<Object_8>"
  Bus Selector1/9 -> Matrix Concatenate/9  "<Object_9>"
  Bus Selector1/10 -> Matrix Concatenate/10  "<Object_10>"

== system controller_dev_sg_HIL_noTP/UDP to Object Detection/Prepare Object List6 ==
  Objects : Inport
  Bus Selector1 : BusSelector  OutputSignals=Object_1,Object_2,Object_3,Object_4,Object_5,Object_6,Object_7,Object_8,Object_9,Object_10
  Byte Pack : etargetslib/Byte Pack  datatypes={['double']}  byteAlign=1
  Data Type Conversion4 : DataTypeConversion
  Matrix Concatenate : Concatenate  NumInputs=10  Mode=Multidimensional array
  ObjList_Package : Outport
  wires:
  Byte Pack/1 -> ObjList_Package/1
  Data Type Conversion4/1 -> Byte Pack/1
  Objects/1 -> Bus Selector1/1
  Matrix Concatenate/1 -> Data Type Conversion4/1
  Bus Selector1/1 -> Matrix Concatenate/1  "<Object_1>"
  Bus Selector1/2 -> Matrix Concatenate/2  "<Object_2>"
  Bus Selector1/3 -> Matrix Concatenate/3  "<Object_3>"
  Bus Selector1/4 -> Matrix Concatenate/4  "<Object_4>"
  Bus Selector1/5 -> Matrix Concatenate/5  "<Object_5>"
  Bus Selector1/6 -> Matrix Concatenate/6  "<Object_6>"
  Bus Selector1/7 -> Matrix Concatenate/7  "<Object_7>"
  Bus Selector1/8 -> Matrix Concatenate/8  "<Object_8>"
  Bus Selector1/9 -> Matrix Concatenate/9  "<Object_9>"
  Bus Selector1/10 -> Matrix Concatenate/10  "<Object_10>"
